simulink model "Code_of_Section_IV_B"  (R2020a)
settings: Solver=FixedStepAuto  StartTime=0.0  StopTime=4  FixedStep=0.0001  RelTol=1e-5  EnableMultiTasking=on
settings Model: Creator=13018  LastModifiedBy=Administrator
settings DataIOCC: ReturnWorkspaceOutputs=off
settings OptimizationCC: LifeSpan=inf
settings DebuggingCC: SFUnexpectedBacktrackingDiag=warning  SFNoUnconditionalDefaultTransitionDiag=warning  ArithmeticOperatorsInVariantConditions=warning
settings SFSimCC: SimUseLocalCustomCode=off  CustomCodeUndefinedFunction=UseInterfaceOnly
settings RTWCC: RTWUseLocalCustomCode=off
settings CodeAppCC: StateflowObjectComments=on
settings GRTTargetCC: TargetLangStandard=C89/C90 (ANSI)
settings ConfigComp: CovMetricSettings=dw  CovHtmlReporting=on  CovSaveCumulativeToWorkspaceVar=on  CovSaveSingleToWorkspaceVar=on  CovExternalEMLEnable=off

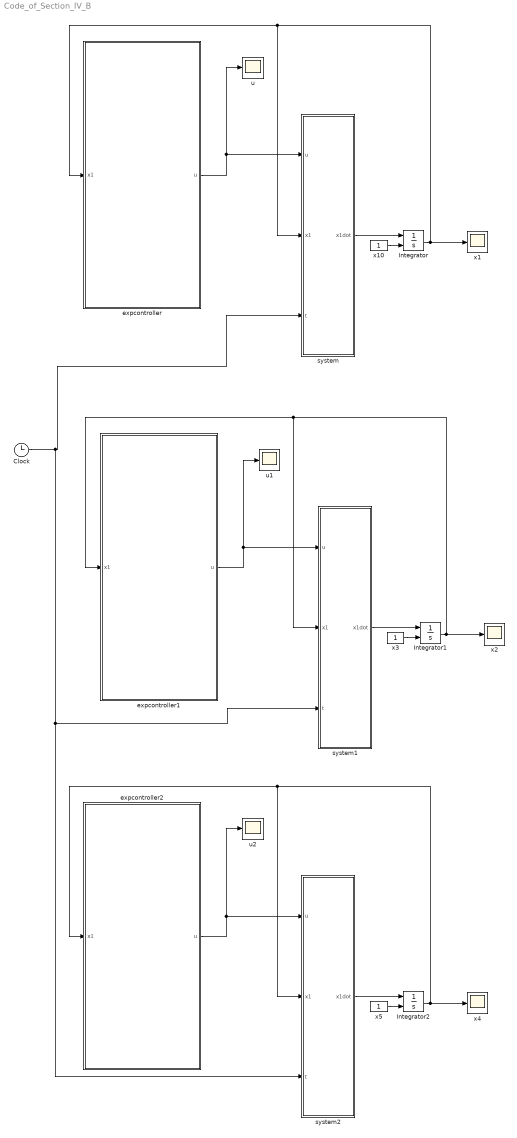
== system Code_of_Section_IV_B ==
  Clock : Clock
  Integrator : Integrator  InitialConditionSource=external
  Integrator1 : Integrator  InitialConditionSource=external
  Integrator2 : Integrator  InitialConditionSource=external
  expcontroller : MATLAB Function  TreatAsAtomicUnit=on
  expcontroller1 : MATLAB Function  TreatAsAtomicUnit=on
  expcontroller2 : MATLAB Function  TreatAsAtomicUnit=on
  system : MATLAB Function  TreatAsAtomicUnit=on
  system1 : MATLAB Function  TreatAsAtomicUnit=on
  system2 : MATLAB Function  TreatAsAtomicUnit=on
  u : Scope
  u1 : Scope
  u2 : Scope
  x1 : Scope
  x10 : Constant  VectorParams1D=off  SampleTime=-1
  x2 : Scope
  x3 : Constant  VectorParams1D=off  SampleTime=-1
  x4 : Scope
  x5 : Constant  VectorParams1D=off  SampleTime=-1
  wires:
  system/1(x1dot) -> Integrator/1
  x10/1 -> Integrator/2
  Integrator/1 -> system/2(x1), expcontroller/1(x1), x1/1
  expcontroller/1(u) -> system/1(u), u/1
  x3/1 -> Integrator1/2
  system1/1(x1dot) -> Integrator1/1
  expcontroller1/1(u) -> u1/1, system1/1(u)
  Integrator1/1 -> system1/2(x1), expcontroller1/1(x1), x2/1
  x5/1 -> Integrator2/2
  system2/1(x1dot) -> Integrator2/1
  expcontroller2/1(u) -> u2/1, system2/1(u)
  Integrator2/1 -> system2/2(x1), expcontroller2/1(x1), x4/1
  Clock/1 -> system1/3(t), system2/3(t), system/3(t)

== matlab function Code_of_Section_IV_B/system1 ==
  data: u input; x1 input; x1dot output; t input
function x1dot  = fcn(u,x1,t)
x1dot=0.5*sin(10*x1)+0.5*cos(10*t)+u;
end

== matlab function Code_of_Section_IV_B/expcontroller2 ==
  data: u output; x1 input
function u   = fcn(x1)
Tc=1;
x1s=0.1;
x1c=1;

u=-log(x1c/x1s)/(Tc)*x1-1/x1s*x1;

end

== matlab function Code_of_Section_IV_B/system2 ==
  data: u input; x1 input; x1dot output; t input
function x1dot  = fcn(u,x1,t)
x1dot=0.5+0.5*cos(x1*t)+u;
end

== matlab function Code_of_Section_IV_B/expcontroller1 ==
  data: u output; x1 input
function u   = fcn(x1)
Tc=1;
x1s=0.1;
x1c=1;

u=-log(x1c/x1s)/(Tc)*x1-1/x1s*x1;
end

== matlab function Code_of_Section_IV_B/system ==
  data: u input; x1 input; x1dot output; t input
function x1dot  = fcn(u,x1,t)
x1dot=cos(10*t)*exp(-t)+u;
end

== matlab function Code_of_Section_IV_B/expcontroller ==
  data: u output; x1 input
function u   = fcn(x1)
Tc=1;
x1s=0.1;
x1c=1;

u=-log(x1c/x1s)/(Tc)*x1-1/x1s*x1;

end
